simulink library "PowerManagementSystem"  (R2013a)
settings: Solver=ode3  StartTime=0.0  StopTime=10.0  RelTol=1e-3
settings Model: Creator=torstebo  LastModifiedBy=torstebo

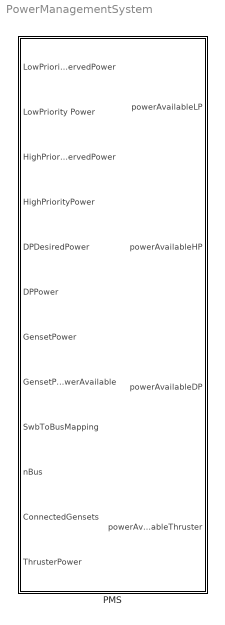
== system PowerManagementSystem ==
  PMS : Subsystem

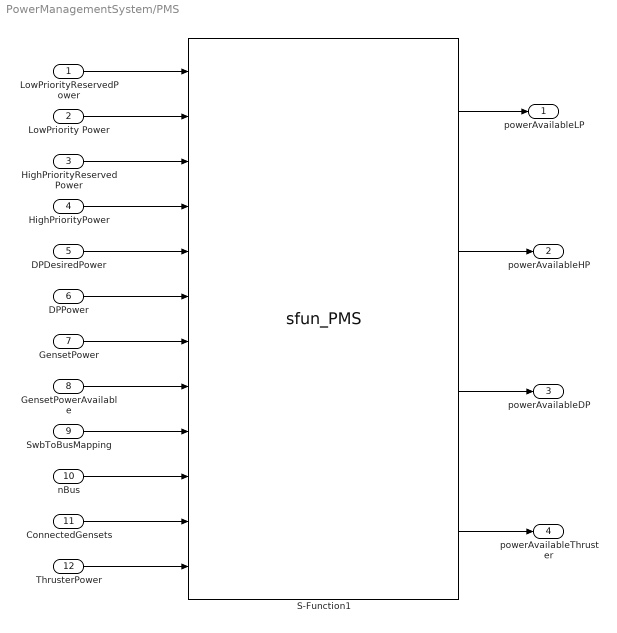
== system PowerManagementSystem/PMS ==
  LowPriorityReservedPower : Inport
  LowPriority Power : Inport  Port=2
  HighPriorityReservedPower : Inport  Port=3
  HighPriorityPower : Inport  Port=4
  DPDesiredPower : Inport  Port=5
  DPPower : Inport  Port=6
  GensetPower : Inport  Port=7
  GensetPowerAvailable : Inport  Port=8
  SwbToBusMapping : Inport  Port=9
  nBus : Inport  Port=10
  ConnectedGensets : Inport  Port=11
  ThrusterPower : Inport  Port=12
  S-Function1 : S-Function  FunctionName=sfun_PMS  Parameters=TSample,NSwitchboard,NGenerators, GeneratorRatedPower, rampTimePowerAvaialble, thrusterRatedPower,FlrRestoreTime,FlrRampTime,nThrusterPerSwitchboard  EnableBusSupport=off
  powerAvailableLP : Outport
  powerAvailableHP : Outport  Port=2
  powerAvailableDP : Outport  Port=3
  powerAvailableThruster : Outport  Port=4
  wires:
  DPDesiredPower/1 -> S-Function1/5
  ThrusterPower/1 -> S-Function1/12
  GensetPowerAvailable/1 -> S-Function1/8
  S-Function1/4 -> powerAvailableThruster/1
  S-Function1/1 -> powerAvailableLP/1
  S-Function1/2 -> powerAvailableHP/1
  HighPriorityReservedPower/1 -> S-Function1/3
  S-Function1/3 -> powerAvailableDP/1
  HighPriorityPower/1 -> S-Function1/4
  LowPriority Power/1 -> S-Function1/2
  LowPriorityReservedPower/1 -> S-Function1/1
  SwbToBusMapping/1 -> S-Function1/9
  nBus/1 -> S-Function1/10
  ConnectedGensets/1 -> S-Function1/11
  GensetPower/1 -> S-Function1/7
  DPPower/1 -> S-Function1/6
